simulink model "simple_control_system_controlled_discreet"  (R2016b)
settings: Solver=VariableStepAuto  StartTime=0.0  StopTime=0.2  RelTol=1e-3
values from neighbouring files (symbols this model uses):
  Kp1 = 0.1    [simple_control_system_matlab.m]
  Ks = 100    [simulink_parameter.m]
  taua = 1e-3    (= 0.001)    [simulink_parameter.m]
  taup = 100e-3    (= 0.1)    [simulink_parameter.m]
  taus = 100e-6    (= 0.0001)    [simulink_parameter.m]
  Ts = 1/fs    (= 0.001)    [simple_control_system_matlab.m]
settings Model: Creator=lapmint  LastModifiedBy=lapmint

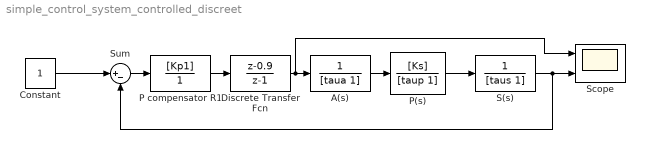
== system simple_control_system_controlled_discreet ==
  A(s) : TransferFcn  Denominator=[taua 1]
  Constant : Constant
  Discrete Transfer Fcn : DiscreteTransferFcn  Numerator=[1 -0.9]  Denominator=[1 -1]  SampleTime=Ts
  P compensator R1 : TransferFcn  Numerator=[Kp1]  Denominator=[0 1]
  P(s) : TransferFcn  Numerator=[Ks]  Denominator=[taup 1]
  S(s) : TransferFcn  Denominator=[taus 1]
  Scope : Scope  NumInputPorts=2
  Sum : Sum  Inputs=|+-
  wires:
  A(s)/1 -> P(s)/1
  P(s)/1 -> S(s)/1
  Constant/1 -> Sum/1
  P compensator R1/1 -> Discrete Transfer Fcn/1
  Discrete Transfer Fcn/1 -> Scope/1, A(s)/1
  Sum/1 -> P compensator R1/1
  S(s)/1 -> Scope/2, Sum/2
